simulink model "statespacesSYSTEM"  (R2014a)
settings: Solver=ode45  StartTime=0.0  StopTime=20  RelTol=1e-3
values from neighbouring files (symbols this model uses):
  A = [-CT,-KT;eye(6),zeros(6)]    [PARAMETER.m]
  B = [zeros(6,2);QT]    [PARAMETER.m]
  D = zeros(12,2)    [PARAMETER.m]
  H = [0 0 0 0 0 0 0 0 0 -1 1 0;0 0 0 0 0 0 -1 0 0 0 1 0;0 0 0 0 0 0 0 -1 0 0 1 0;0 0 0 ch/mh -ch/mh 0 0 0 0 kh/mh -kh/mh 0]    [PARAMETER.m]
  J = lqr(A,B,Q,R)    [PARAMETER.m]
libraries: simulink_extras x1, simulink x1
settings Model: Creator=Administrator  LastModifiedBy=Administrator

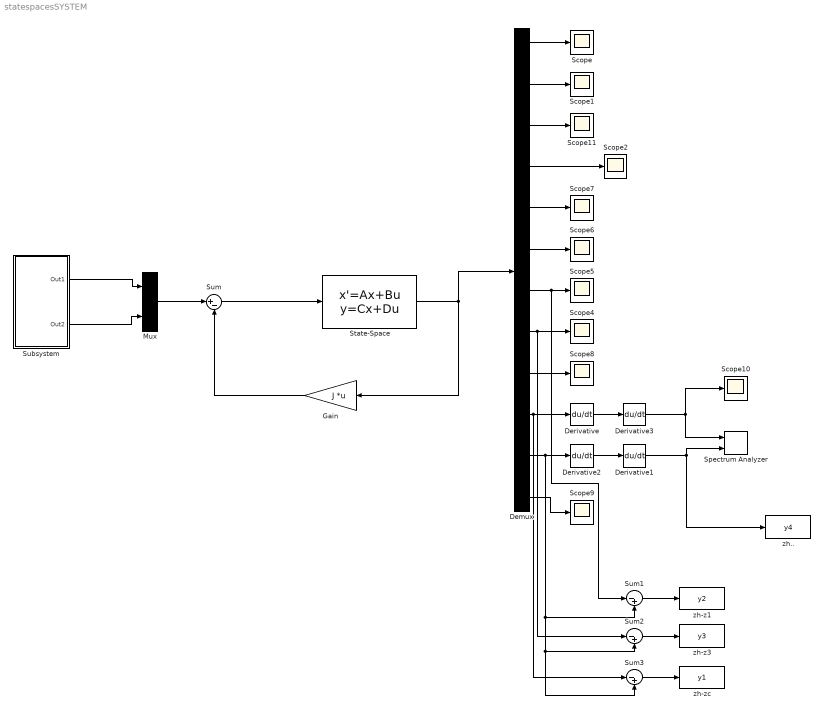
== system statespacesSYSTEM ==
  Demux : Demux  Outputs=12
  Derivative{,1..3} (4 alike) : Derivative
  Gain : Gain  Gain=J  Multiplication=Matrix(K*u)
  Mux : Mux  Inputs=2
  Scope{,1..2,4..11} (11 alike) : Scope
      Scope10 settings: SaveName=ScopeData10
      Scope11 settings: SaveName=ScopeData12
      Scope2 settings: SaveName=ScopeData2
      Scope4 settings: SaveName=ScopeData4
      Scope5 settings: SaveName=ScopeData5
      Scope6 settings: SaveName=ScopeData6
      Scope7 settings: SaveName=ScopeData7
      Scope8 settings: SaveName=ScopeData8
      Scope9 settings: SaveName=ScopeData9
  Spectrum Analyzer : simulink_extras/Additional Sinks/Spectrum Analyzer  npts=256  fftpts=256  HowOften=64  sampleT=0.1
  State-Space : StateSpace  A=A  B=B  C=H  D=D  X0=0
  Subsystem : Subsystem
  Sum : Sum  Inputs=|+-
  Sum1 : Sum  Inputs=|-+
  Sum2 : Sum  Inputs=|-+
  Sum3 : Sum  Inputs=|-+
  zh-z1 : ToWorkspace  VariableName=y2  SaveFormat=Timeseries  SampleTime=-1
  zh-z3 : ToWorkspace  VariableName=y3  SaveFormat=Timeseries  SampleTime=-1
  zh-zc : ToWorkspace  VariableName=y1  SaveFormat=Timeseries  SampleTime=-1
  zh.. : ToWorkspace  VariableName=y4  SaveFormat=Timeseries  SampleTime=-1
  wires:
  Subsystem/1(Out1) -> Mux/1
  Subsystem/2(Out2) -> Mux/2
  Demux/2 -> Scope1/1
  Demux/1 -> Scope/1
  Mux/1 -> Sum/1
  Demux/3 -> Scope11/1
  Demux/4 -> Scope2/1
  State-Space/1 -> Gain/1, Demux/1
  Demux/5 -> Scope7/1
  Derivative2/1 -> Derivative1/1
  Derivative/1 -> Derivative3/1
  Derivative3/1 -> Spectrum Analyzer/1, Scope10/1
  Derivative1/1 -> zh../1, Spectrum Analyzer/2
  Gain/1 -> Sum/2
  Sum/1 -> State-Space/1
  Demux/10 -> Derivative/1, Sum3/1
  Demux/11 -> Sum3/2, Sum2/2, Sum1/2, Derivative2/1
  Demux/6 -> Scope6/1
  Demux/7 -> Sum1/1, Scope5/1
  Demux/9 -> Scope8/1
  Demux/12 -> Scope9/1
  Sum1/1 -> zh-z1/1
  Demux/8 -> Scope4/1, Sum2/1
  Sum2/1 -> zh-z3/1
  Sum3/1 -> zh-zc/1

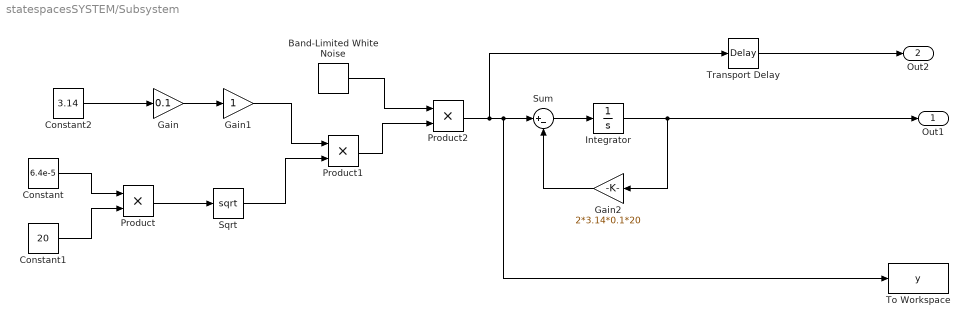
== system statespacesSYSTEM/Subsystem ==
  Band-Limited White Noise : simulink/Sources/Band-Limited White Noise  Cov=[0.1]  Ts=0.1  seed=[23341]
  Constant : Constant  Value=6.4e-5
  Constant1 : Constant  Value=20
  Constant2 : Constant  Value=3.14
  Gain : Gain  Gain=0.1
  Gain1 : Gain
  Gain2 : Gain  Gain=2*3.14*0.1*20
  Integrator : Integrator
  Product : Product
  Product1 : Product
  Product2 : Product
  Sqrt : Sqrt  SaturateOnIntegerOverflow=on
  Sum : Sum  Inputs=|+-
  To Workspace : ToWorkspace  VariableName=y  SaveFormat=Timeseries  SampleTime=-1
  Transport Delay : TransportDelay
  Out1 : Outport
  Out2 : Outport  Port=2
  wires:
  Gain2/1 -> Sum/2
  Product/1 -> Sqrt/1
  Gain/1 -> Gain1/1
  Product1/1 -> Product2/2
  Constant/1 -> Product/1
  Sqrt/1 -> Product1/2
  Constant1/1 -> Product/2
  Constant2/1 -> Gain/1
  Band-Limited White Noise/1 -> Product2/1
  Integrator/1 -> Out1/1, Gain2/1
  Sum/1 -> Integrator/1
  Gain1/1 -> Product1/1
  Transport Delay/1 -> Out2/1
  Product2/1 -> To Workspace/1, Sum/1, Transport Delay/1
